simulink model "sistemaControl"  (R2024b)
settings: Solver=VariableStepAuto  StartTime=0.0  StopTime=10.0  RelTol=1e-3
settings Model: Creator=estel  LastModifiedBy=estel

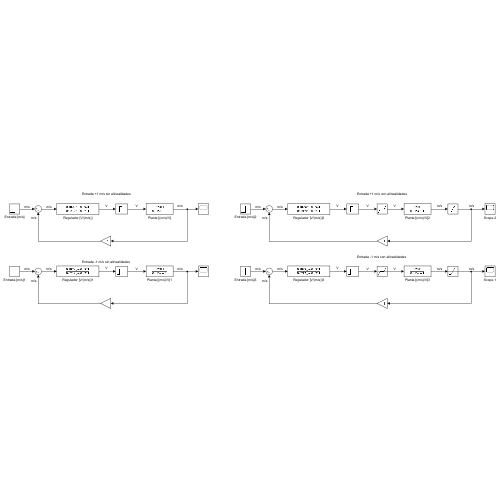
[thumbnail: Simulink's stored preview of the top-level diagram]
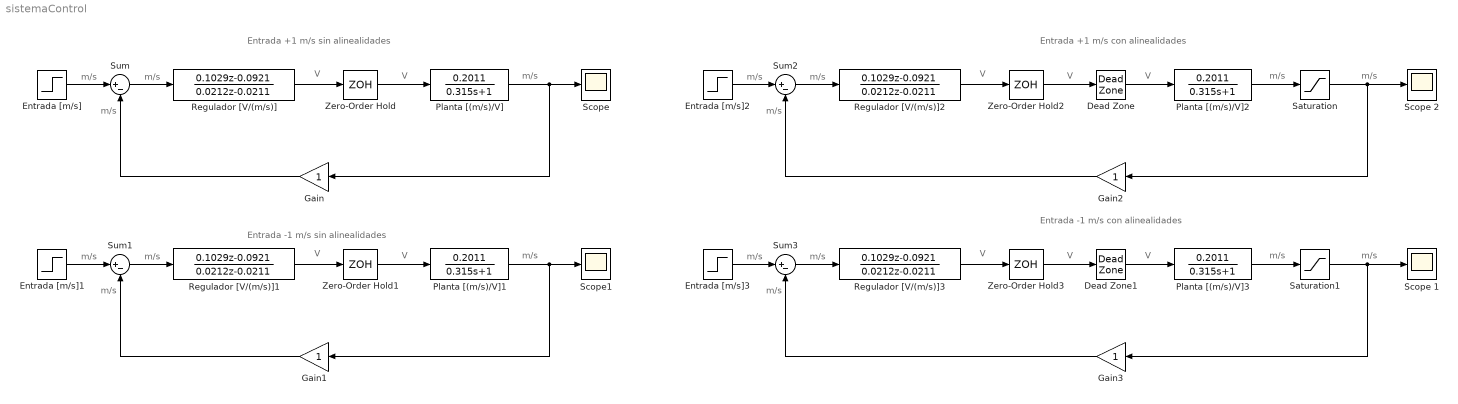
== system sistemaControl ==
  note: Entrada +1 m/s sin alinealidades
  note: m/s
  note: m/s
  note: m/s
  note: m/s
  note: V
  note: V
  note: m/s
  note: m/s
  note: m/s
  note: m/s
  note: V
  note: V
  note: Entrada -1 m/s sin alinealidades
  note: Entrada +1 m/s con alinealidades
  note: m/s
  note: m/s
  note: m/s
  note: m/s
  note: V
  note: V
  note: m/s
  note: V
  note: Entrada -1 m/s con alinealidades
  note: m/s
  note: m/s
  note: m/s
  note: m/s
  note: V
  note: V
  note: m/s
  note: V
  Dead Zone : DeadZone  LowerValue=-0.19  UpperValue=0.19
  Dead Zone1 : DeadZone  LowerValue=-0.19  UpperValue=0.19
  Entrada [m/s] : Step  SampleTime=0
  Entrada [m/s]1 : Step  After=-1  SampleTime=0
  Entrada [m/s]2 : Step  SampleTime=0
  Entrada [m/s]3 : Step  After=-1  SampleTime=0
  Gain{,1..3} (4 alike) : Gain
  Planta [(m/s)/V]{,1..3} (4 alike) : TransferFcn  Numerator=[0.2011]  Denominator=[0.315 1]
  Regulador [V/(m/s)]{,1..3} (4 alike) : DiscreteTransferFcn  Numerator=[0.1029 -0.0921]  Denominator=[0.0212 -0.0211]
  Saturation : Saturate  UpperLimit=10  LowerLimit=-10
  Saturation1 : Saturate  UpperLimit=10  LowerLimit=-10
  Scope : Scope
  Scope 1 : Scope
  Scope 2 : Scope
  Scope1 : Scope
  Sum{,1..3} (4 alike) : Sum  Inputs=|+-
  Zero-Order Hold{,1..3} (4 alike) : ZeroOrderHold  SampleTime=-1
  wires:
  Entrada [m/s]/1 -> Sum/1
  Sum/1 -> Regulador [V/(m/s)]/1
  Regulador [V/(m/s)]/1 -> Zero-Order Hold/1
  Zero-Order Hold/1 -> Planta [(m/s)/V]/1
  Planta [(m/s)/V]/1 -> Gain/1, Scope/1
  Gain/1 -> Sum/2
  Gain1/1 -> Sum1/2
  Planta [(m/s)/V]1/1 -> Scope1/1, Gain1/1
  Zero-Order Hold1/1 -> Planta [(m/s)/V]1/1
  Regulador [V/(m/s)]1/1 -> Zero-Order Hold1/1
  Sum1/1 -> Regulador [V/(m/s)]1/1
  Entrada [m/s]1/1 -> Sum1/1
  Gain2/1 -> Sum2/2
  Regulador [V/(m/s)]2/1 -> Zero-Order Hold2/1
  Sum2/1 -> Regulador [V/(m/s)]2/1
  Entrada [m/s]2/1 -> Sum2/1
  Planta [(m/s)/V]2/1 -> Saturation/1
  Saturation/1 -> Gain2/1, Scope 2/1
  Dead Zone/1 -> Planta [(m/s)/V]2/1
  Zero-Order Hold2/1 -> Dead Zone/1
  Zero-Order Hold3/1 -> Dead Zone1/1
  Dead Zone1/1 -> Planta [(m/s)/V]3/1
  Saturation1/1 -> Scope 1/1, Gain3/1
  Planta [(m/s)/V]3/1 -> Saturation1/1
  Entrada [m/s]3/1 -> Sum3/1
  Sum3/1 -> Regulador [V/(m/s)]3/1
  Regulador [V/(m/s)]3/1 -> Zero-Order Hold3/1
  Gain3/1 -> Sum3/2
